simulink model "LoadFlow116BusNetwork_original"  (R2024a)
settings: Solver=FixedStepDiscrete  StartTime=0.0  StopTime=4.5  FixedStep=75e-6  RelTol=1e-3  EnableMultiTasking=on
undefined symbols (not defined in the file or in its folder): D1, D11, Delta
libraries: spsSeriesRLCBranchLib x164, spsLoadFlowBusLib x116, spsDistributedParametersLineLib x79, spsThreePhaseSeriesRLCLoadLib x60, spsThreePhaseTransformerTwoWindingsLib x52, spsThreePhaseParallelRLCLoadLib x44, spsThreePhaseVIMeasurementLib x44, spsSynchronousMachinepuStandardLib x28, spsExcitationSystemLib x28, spsHydraulicTurbineandGovernorLib x28, spsGenericPowerSystemStabilizerLib x28, spsMultiBandPowerSystemStabilizerLib x28
(part 5 of 15)

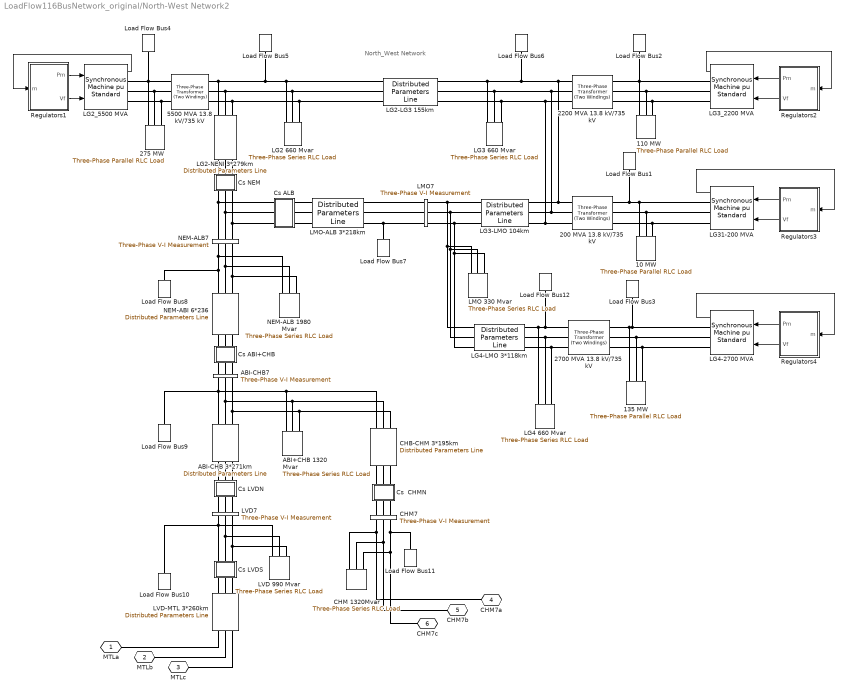
== system LoadFlow116BusNetwork_original/North-West Network2 ==
  note: North_West Network
  10 MW : spsThreePhaseParallelRLCLoadLib/Three-Phase Parallel RLC Load  LConnTagsString=A|B|C  Configuration=Y (grounded)  NominalVoltage=(13800)*1  Vabc=[1e3 1e3 1e3]  Vabcp=[1e3 1e3 1e3]  NominalFrequency=60  UnbalancedPower=off  ActivePower=10000000  InductivePower=0  CapacitivePower=0  Pabc=[10e3 9e3 11e3]  QLabc=[100 90 110]  QCabc=[100 90 110]  Pabcp=[10e3 9e3 11e3]  QLabcp=[100 90 110]  QCabcp=[100 90 110]  Measurements=None  LoadType=constant PQ
  110 MW : spsThreePhaseParallelRLCLoadLib/Three-Phase Parallel RLC Load  LConnTagsString=A|B|C  Configuration=Y (grounded)  NominalVoltage=(13800)*1  Vabc=[1e3 1e3 1e3]  Vabcp=[1e3 1e3 1e3]  NominalFrequency=60  UnbalancedPower=off  ActivePower=110000000  InductivePower=0  CapacitivePower=0  Pabc=[10e3 9e3 11e3]  QLabc=[100 90 110]  QCabc=[100 90 110]  Pabcp=[10e3 9e3 11e3]  QLabcp=[100 90 110]  QCabcp=[100 90 110]  Measurements=None  LoadType=constant PQ
  135 MW : spsThreePhaseParallelRLCLoadLib/Three-Phase Parallel RLC Load  LConnTagsString=A|B|C  Configuration=Y (grounded)  NominalVoltage=(13800)*1  Vabc=[1e3 1e3 1e3]  Vabcp=[1e3 1e3 1e3]  NominalFrequency=60  UnbalancedPower=off  ActivePower=135000000  InductivePower=0  CapacitivePower=0  Pabc=[10e3 9e3 11e3]  QLabc=[100 90 110]  QCabc=[100 90 110]  Pabcp=[10e3 9e3 11e3]  QLabcp=[100 90 110]  QCabcp=[100 90 110]  Measurements=None  LoadType=constant PQ
  200 MVA 13.8 kV/735 kV : spsThreePhaseTransformerTwoWindingsLib/Three-Phase Transformer (Two Windings)  Winding1Connection=Delta (D1)  Winding2Connection=Yg  CoreType=Three single-phase transformers  SetSaturation=off  Hysteresis=off  DataFile='basic_model'  SetInitialFlux=off  Measurements=None  UNITS=pu  NominalPower=[ 200e6 60 ]  Winding1="[ 13.8e3 0.002  0.0]"  Winding2=[ 735e3 0.002 0.12]  Rm=500  Lm=500  L0=0.5  Saturation="[ 0,0  ;  0.005,1.2  ;  1.0,1.4 ]"  InitialFluxes=[ 0.8 , -0.8 , 0.7 ]  BreakLoop=off  DiscreteSolver=Trapezoidal iterative  DataType=off  TransfoNumber=0
  2200 MVA 13.8 kV/735 kV : spsThreePhaseTransformerTwoWindingsLib/Three-Phase Transformer (Two Windings)  Winding1Connection=Delta (D1)  Winding2Connection=Yg  CoreType=Three single-phase transformers  SetSaturation=off  Hysteresis=off  DataFile='basic_model'  SetInitialFlux=off  Measurements=None  UNITS=pu  NominalPower=[ 2200e6 60 ]  Winding1="[ 13.8e3 0.002  0.0]"  Winding2=[ 735e3 0.002 0.12]  Rm=500  Lm=500  L0=0.5  Saturation="[ 0,0  ;  0.005,1.2  ;  1.0,1.4 ]"  InitialFluxes=[ 0.8 , -0.8 , 0.7 ]  BreakLoop=off  DiscreteSolver=Trapezoidal iterative  DataType=off  TransfoNumber=0
  2700 MVA 13.8 kV/735 kV : spsThreePhaseTransformerTwoWindingsLib/Three-Phase Transformer (Two Windings)  Winding1Connection=Delta (D1)  Winding2Connection=Yg  CoreType=Three single-phase transformers  SetSaturation=off  Hysteresis=off  DataFile='basic_model'  SetInitialFlux=off  Measurements=None  UNITS=pu  NominalPower=[ 2700e6 60 ]  Winding1="[ 13.8e3 0.002  0.0]"  Winding2=[ 735e3 0.002 0.12]  Rm=500  Lm=500  L0=0.5  Saturation="[ 0,0  ;  0.005,1.2  ;  1.0,1.4 ]"  InitialFluxes=[ 0.8 , -0.8 , 0.7 ]  BreakLoop=off  DiscreteSolver=Trapezoidal iterative  DataType=off  TransfoNumber=0
  275 MW : spsThreePhaseParallelRLCLoadLib/Three-Phase Parallel RLC Load  LConnTagsString=A|B|C  Configuration=Y (grounded)  NominalVoltage=(13800)*1  Vabc=[1e3 1e3 1e3]  Vabcp=[1e3 1e3 1e3]  NominalFrequency=60  UnbalancedPower=off  ActivePower=275000000  InductivePower=0  CapacitivePower=0  Pabc=[10e3 9e3 11e3]  QLabc=[100 90 110]  QCabc=[100 90 110]  Pabcp=[10e3 9e3 11e3]  QLabcp=[100 90 110]  QCabcp=[100 90 110]  Measurements=None  LoadType=constant PQ
  5500 MVA 13.8 kV/735 kV : spsThreePhaseTransformerTwoWindingsLib/Three-Phase Transformer (Two Windings)  Winding1Connection=Delta (D1)  Winding2Connection=Yg  CoreType=Three single-phase transformers  SetSaturation=off  Hysteresis=off  DataFile='basic_model'  SetInitialFlux=off  Measurements=None  UNITS=pu  NominalPower=[ 5500e6 60 ]  Winding1="[ 13.8e3 0.002  0.0]"  Winding2=[ 735e3 0.002 0.12]  Rm=500  Lm=500  L0=0.5  Saturation="[ 0,0  ;  0.005,1.2  ;  1.0,1.4 ]"  InitialFluxes=[ 0.8 , -0.8 , 0.7 ]  BreakLoop=off  DiscreteSolver=Trapezoidal iterative  DataType=off  TransfoNumber=0
  ABI+CHB 1320 Mvar : spsThreePhaseSeriesRLCLoadLib/Three-Phase Series RLC Load  LConnTagsString=A|B|C  Configuration=Y (grounded)  NominalVoltage=735e3  Vabc=[1e3 1e3 1e3]  Vabcp=[1e3 1e3 1e3]  NominalFrequency=60  UnbalancedPower=off  ActivePower=4400000  InductivePower=1320e6  CapacitivePower=0  Pabc=[10e3 9e3 11e3]  QLabc=[100 90 110]  QCabc=[100 90 110]  Pabcp=[10e3 9e3 11e3]  QLabcp=[100 90 110]  QCabcp=[100 90 110]  Measurements=None  LoadType=constant Z
  ABI-CHB 3*271km : spsDistributedParametersLineLib/Distributed Parameters Line  Phases=3  Length=271  Frequency=60  Resistance="[0.01273  0.3864]/3"  Inductance="[0.9337e-3  4.1264e-3]/3"  Capacitance=[12.74e-9 7.751e-9]*3  x1=[-0.001575 3.49112965554761e-09 -103484.456536088 -819305.847115511;-0.0015 3.54940703648419e-09 -80280.8596537815 -821903.919579572;-0.001425 3.60484707574356e-09 -57013.0874806064 -823844.974625874;-0.00135 3.65740545540659e-09 -33699.7399176288 -825127.46060471;-0.001275 3.70704016110874e-09 -10359.4532981844 -825750.352316412;-0.0012 3.75371151562572e-09 12989.1145097218 -825713.151830876;-0.001125 3.79738221059082e-09 36327.2990182289 -825015.888885602;-0.00105 3.83801733631867e-09 59636.4440397272 -823659.120861919;-0.000975 3.87558440971151e-09 82897.9166003282 -821643.932339426;-0.0009 3.91005340022564e-09 106093.12183478 -818971.934228995;-0.000825 3.94139675387747e-09 129203.517850916 -815645.262485032;-0.00075 3.96958941526963e-09 152210.630551762 -811666.57639803;-0.000675 3.99460884761998e-09 175096.068403445 -807039.05646877;-0.0006 4.01643505077712e-09 197841.537137107 -801766.40186588;-0.000525 4.03505057720817e-09 220428.854373058 -795852.827468776;-0.00045 4.05044054594615e-09 242839.964155498 -789303.06049835;-0.000375 4.06259265448552e-09 265056.951386168 -782122.336738104;-0.0003 4.07149718861665e-09 287062.056145408 -774316.396348742;-0.000225 4.07714703019119e-09 308837.687889161 -765891.479279577;-0.00015 4.07953766281224e-09 330366.439510591 -756854.320280409;-7.5e-05 4.07866717544465e-09 351631.101255053 -747212.143517868]  x2=[-0.001575 8.85627598143127e-09 -329701.158011524 -748762.187115691;-0.0015 9.00536203977742e-09 -308401.44100994 -757783.743021183;-0.001425 9.14724934949562e-09 -286855.192615113 -766199.538196984;-0.00135 9.28182448804145e-09 -265079.63656834 -774002.845185196;-0.001275 9.40897987810821e-09 -243092.179915949 -781187.426141608;-0.0012 9.52861387362263e-09 -220910.399094369 -787747.537822131;-0.001125 9.64063084099916e-09 -198552.025879795 -793677.93617386;-0.00105 9.74494123558799e-09 -176034.93321368 -798973.880527091;-0.000975 9.84146167325569e-09 -153377.12091538 -803631.13738494;-0.0009 9.93011499704121e-09 -130596.701293368 -807645.983807531;-0.000825 1.00108303388339e-08 -107711.884666539 -811015.210388065;-0.00075 1.00835431760247e-08 -84740.9648071545 -813736.123818364;-0.000675 1.01481953830838e-08 -61702.3043170834 -815806.549041862;-0.0006 1.02047352780264e-08 -38614.3199490181 -817224.830992315;-0.000525 1.02531176637254e-08 -15495.4678844046 -817989.835916832;-0.00045 1.02933038640419e-08 7635.77102014722 -818100.952282181;-0.000375 1.03252617547424e-08 30760.9060061767 -817558.09126364;-0.0003 1.03489657891779e-08 53861.4511946025 -816361.686816001;-0.000225 1.0364397018706e-08 76918.9403630512 -814512.695326674;-0.00015 1.0371543107838e-08 99914.9417074729 -812012.594851165;-7.5e-05 1.03703983440995e-08 122831.072576243 -808863.383931542]  x3=[-0.001575 -2.33509162895543e-12 -747.841433917336 -1501.46113433937;-0.0015 -8.83661713204438e-13 -705.09503694803 -1522.0023117976;-0.001425 5.68474588199612e-13 -661.784997794503 -1541.32682389519;-0.00135 2.02015645971581e-12 -617.94593783939 -1559.41922291285;-0.001275 3.47022344906753e-12 -573.612901356457 -1576.26504606363;-0.0012 4.91751639489027e-12 -528.821327496752 -1591.85082705425;-0.001125 6.36087835334746e-12 -483.607021959084 -1606.16410684986;-0.00105 7.79915552297369e-12 -438.006128367497 -1619.19344363358;-0.000975 9.23119816700594e-12 -392.055099378611 -1630.92842195296;-0.0009 1.06558615324655e-11 -345.790667541927 -1641.35966104587;-0.000825 1.20720067652562e-11 -299.249815936384 -1650.47882233938;-0.00075 1.34785018205467e-11 -252.469748606657 -1658.27861611549;-0.000675 1.48742223677098e-11 -205.487860822811 -1664.75280733839;-0.0006 1.62580526890954e-11 -158.341709187093 -1669.89622063867;-0.000525 1.76288865719179e-11 -111.06898161176 -1673.70474445044;-0.00045 1.89856281925458e-11 -63.7074671919388 -1676.17533429805;-0.000375 2.03271929924864e-11 -16.2950259976015 -1677.30601522975;-0.0003 2.16525085453653e-11 31.1304411911961 -1677.09588339653;-0.000225 2.29605154142075e-11 78.5310231816171 -1675.54510677455;-0.00015 2.42501679983353e-11 125.868828673672 -1672.65492503091;-7.5e-05 2.55204353692052e-11 173.106016549942 -1668.42764853267]  x4=[-0.001575 3.79881308339713e-11 -7080.29438162328 -14859.1258761626;-0.0015 3.76223755888515e-11 -6657.38891399992 -15053.3510061731;-0.001425 3.72265455923276e-11 -6229.16163154018 -15235.5427177132;-0.00135 3.68009572648424e-11 -5795.95485258156 -15405.5553695164;-0.001275 3.63459508151933e-11 -5358.11487599487 -15563.2530560702;-0.0012 3.58618899685742e-11 -4915.99170435821 -15708.5097162566;-0.001125 3.53491616758195e-11 -4469.93876417028 -15841.2092341242;-0.00105 3.48081758040815e-11 -4020.31262332663 -15961.2455317086;-0.000975 3.42393648091886e-11 -3567.47270608474 -16068.5226538302;-0.0009 3.36431833899472e-11 -3111.78100574577 -16162.9548447989;-0.000825 3.30201081246617e-11 -2653.60179528266 -16244.4666169663;-0.00075 3.23706370901661e-11 -2193.30133614586 -16312.9928110687;-0.000675 3.16952894636679e-11 -1731.24758547958 -16368.4786483151;-0.0006 3.09946051077266e-11 -1267.80990198245 -16410.8797741762;-0.000525 3.02691441386956e-11 -803.358750647814 -16440.1622938406;-0.00045 2.95194864789735e-11 -338.265406619711 -16456.3027993103;-0.000375 2.87462313934234e-11 127.098341598809 -16459.2883881121;-0.0003 2.79499970103296e-11 592.360489347724 -16449.116673612;-0.000225 2.71314198272749e-11 1057.14911318487 -16425.795786923;-0.00015 2.6291154202335e-11 1521.09266819587 -16389.3443704049;-7.5e-05 2.54298718309939e-11 1983.82028500141 -16339.7915627626]  x5=0.00153261764655846  V1=ones(3,3)  V2=ones(3,3)  I1=ones(3,3)  I2=ones(3,3)  nHarmo=1  Measurements=None  Decoupling=off  VsMag0=[ 1 1 1]  VrMag0=[ 1 1 1]  VsAngle0=[0 -120 120]  VrAngle0=[0 -120 120]  IsMag0=[ 1 1 1]  IrMag0=[ 1 1 1]  IsAngle0=[0 -120 120]  IrAngle0=[0 -120 120]
      settings: AttributesFormatString=\n  LibrarySourceBlock=sps_lib/Power Grid Elements/Distributed Parameters Line
  ABI-CHB7 : spsThreePhaseVIMeasurementLib/Three-Phase V-I Measurement  VoltageMeasurement=no  SetLabelV=on  LabelV=Vabc_ABI7  Vpu=on  VpuLL=off  CurrentMeasurement=no  SetLabelI=off  LabelI=A1  Ipu=off  Pbase=100e6  Vbase=500e3  OutputType=Magnitude  PhasorSimulation=off  PSBequivalent=0
  CHB-CHM 3*195km : spsDistributedParametersLineLib/Distributed Parameters Line  Phases=3  Length=195  Frequency=60  Resistance="[0.01273  0.3864]/3"  Inductance="[0.9337e-3  4.1264e-3]/3"  Capacitance=[12.74e-9 7.751e-9]*3  x1=[-0.001125 3.79738221059082e-09 0 0;-0.00105 3.83801733631867e-09 0 0;-0.000975 3.87558440971151e-09 0 0;-0.0009 3.91005340022564e-09 0 0;-0.000825 3.94139675387747e-09 0 0;-0.00075 3.96958941526963e-09 0 0;-0.000675 3.99460884761998e-09 175096.068403445 -807039.05646877;-0.0006 4.01643505077712e-09 197841.537137107 -801766.40186588;-0.000525 4.03505057720817e-09 220428.854373058 -795852.827468776;-0.00045 4.05044054594615e-09 242839.964155498 -789303.06049835;-0.000375 4.06259265448552e-09 265056.951386168 -782122.336738104;-0.0003 4.07149718861665e-09 287062.056145408 -774316.396348742;-0.000225 4.07714703019119e-09 308837.687889161 -765891.479279577;-0.00015 4.07953766281224e-09 330366.439510591 -756854.320280409;-7.5e-05 4.07866717544465e-09 351631.101255053 -747212.143517868]  x2=[-0.001125 2.70727178831933e-09 0 0;-0.00105 2.73262221708917e-09 0 0;-0.000975 2.75578822946918e-09 0 0;-0.0009 2.77675130690354e-09 0 0;-0.000825 2.79549469182887e-09 0 0;-0.00075 2.81200340107006e-09 0 0;-0.000675 2.82626423781753e-09 86661.6913681537 -814290.344127287;-0.0006 2.83826580217658e-09 109647.510746712 -811514.902082689;-0.000525 2.8479985002803e-09 132545.679582843 -808090.747441961;-0.00045 2.85545455195872e-09 155337.893430733 -804020.617421931;-0.000375 2.86062799695824e-09 178005.932543363 -799307.765622262;-0.0003 2.86351469970606e-09 200531.6764371 -793955.959424573;-0.000225 2.86411235261617e-09 222897.118376931 -787969.476980854;-0.00015 2.862420477934e-09 245084.379770771 -781353.103793574;-7.5e-05 2.85844042811827e-09 267075.72446134 -774112.128890224]  x3=[-0.001125 1.76155641183731e-11 0 0;-0.00105 1.7454951833372e-11 0 0;-0.000975 1.72803863269451e-11 0 0;-0.0009 1.70920071440872e-11 0 0;-0.000825 1.68899648722348e-11 0 0;-0.00075 1.66744210208886e-11 0 0;-0.000675 1.64455478925056e-11 335.259499976979 -5255.16303225153;-0.0006 1.62035284447626e-11 483.69285157656 -5243.58412650834;-0.000525 1.59485561443032e-11 631.73954651134 -5227.81357984395;-0.00045 1.5680834812083e-11 779.281238518578 -5207.86399899206;-0.000375 1.5400578460439e-11 926.199985027146 -5183.75133134236;-0.0003 1.51080111220104e-11 1072.37834143902 -5155.49485219245;-0.000225 1.48033666706512e-11 1217.69945501268 -5123.11714933941;-0.00015 1.44868886344746e-11 1362.04715827344 -5086.64410502351;-7.5e-05 1.41588300011804e-11 1505.30606187589 -5046.10487523831]  x4=[-0.001125 5.67670866959794e-12 0 0;-0.00105 6.209051937135e-12 0 0;-0.000975 6.73643178355519e-12 0 0;-0.0009 7.25842662947847e-12 0 0;-0.000825 7.7746192002118e-12 0 0;-0.00075 8.28459685931214e-12 0 0;-0.000675 8.78795193844173e-12 265.942029614519 -12956.0177279487;-0.0006 9.2842820632519e-12 632.108856781867 -12943.3211843342;-0.000525 9.77319047503499e-12 997.770385800693 -12920.2779478045;-0.00045 1.02542863478872e-11 1362.63431243951 -12886.9064387702;-0.000375 1.07271851011287e-11 1726.40897005797 -12843.2333339049;-0.0003 1.11915087067318e-11 2088.8035627607 -12789.2935448207;-0.000225 1.16468859915106e-11 2449.52839785513 -12725.1301901594;-0.00015 1.20929529338311e-11 2808.29511742736 -12650.7945611252;-7.5e-05 1.25293529546046e-11 3164.81692885107 -12566.3460804824]  x5=0.0011028060556417  V1=ones(3,3)  V2=ones(3,3)  I1=ones(3,3)  I2=ones(3,3)  nHarmo=1  Measurements=None  Decoupling=off  VsMag0=[ 1 1 1]  VrMag0=[ 1 1 1]  VsAngle0=[0 -120 120]  VrAngle0=[0 -120 120]  IsMag0=[ 1 1 1]  IrMag0=[ 1 1 1]  IsAngle0=[0 -120 120]  IrAngle0=[0 -120 120]
      settings: AttributesFormatString=\n  LibrarySourceBlock=sps_lib/Power Grid Elements/Distributed Parameters Line
  CHM 1320Mvar : spsThreePhaseSeriesRLCLoadLib/Three-Phase Series RLC Load  LConnTagsString=A|B|C  Configuration=Y (grounded)  NominalVoltage=735e3  Vabc=[1e3 1e3 1e3]  Vabcp=[1e3 1e3 1e3]  NominalFrequency=60  UnbalancedPower=off  ActivePower=4400000  InductivePower=1320e6  CapacitivePower=0  Pabc=[10e3 9e3 11e3]  QLabc=[100 90 110]  QCabc=[100 90 110]  Pabcp=[10e3 9e3 11e3]  QLabcp=[100 90 110]  QCabcp=[100 90 110]  Measurements=None  LoadType=constant Z
  CHM7 : spsThreePhaseVIMeasurementLib/Three-Phase V-I Measurement  VoltageMeasurement=no  SetLabelV=on  LabelV=Vabc_CHM7  Vpu=on  VpuLL=off  CurrentMeasurement=no  SetLabelI=off  LabelI=A1  Ipu=off  Pbase=100e6  Vbase=735e3  OutputType=Magnitude  PhasorSimulation=off  PSBequivalent=0
  "Cs  CHMN " : Subsystem  mask{Xc=25/3}
      mask prompts: Xc "Condensator Reactance at  60Hz  (ohm):"
      mask help: Series Compensation
      mask init:
      | Cs=1/Xc/(2*pi*60);
      mask Display: disp('Cs')
  "Cs ABI+CHB " : Subsystem  mask{Xc=25/6}
      mask prompts: Xc "Condensator Reactance at  60Hz  (ohm):"
      mask help: Series Compensation
      mask init:
      | Cs=1/Xc/(2*pi*60);
      mask Display: disp('Cs')
  Cs ALB : Subsystem  mask{Xc=16/3}
      mask prompts: Xc "Reactance @ 60Hz du condensateur (ohm):"
      mask init:
      | Cs=1/Xc/(2*pi*60);
      mask Display: disp('Cs')
  "Cs LVDN " : Subsystem  mask{Xc=34/3}
      mask prompts: Xc "Condensator Reactance at  60Hz  (ohm):"
      mask help: Series Compensation
      mask init:
      | Cs=1/Xc/(2*pi*60);
      mask Display: disp('Cs')
  "Cs LVDS " : Subsystem  mask{Xc=34/3}
      mask prompts: Xc "Condensator Reactance at  60Hz  (ohm):"
      mask help: Series Compensation
      mask init:
      | Cs=1/Xc/(2*pi*60);
      mask Display: disp('Cs')
  "Cs NEM " : Subsystem  mask{Xc=16/3}
      mask prompts: Xc "Condensator Reactance at  60Hz  (ohm):"
      mask help: Series Compensation
      mask init:
      | Cs=1/Xc/(2*pi*60);
      mask Display: disp('Cs')
  LG2 660 Mvar : spsThreePhaseSeriesRLCLoadLib/Three-Phase Series RLC Load  LConnTagsString=A|B|C  Configuration=Y (grounded)  NominalVoltage=735e3  Vabc=[1e3 1e3 1e3]  Vabcp=[1e3 1e3 1e3]  NominalFrequency=60  UnbalancedPower=off  ActivePower=2200000  InductivePower=660e6  CapacitivePower=0  Pabc=[10e3 9e3 11e3]  QLabc=[100 90 110]  QCabc=[100 90 110]  Pabcp=[10e3 9e3 11e3]  QLabcp=[100 90 110]  QCabcp=[100 90 110]  Measurements=None  LoadType=constant Z
  LG2-LG3 155km : spsDistributedParametersLineLib/Distributed Parameters Line  Phases=3  Length=155  Frequency=60  Resistance="[0.01273  0.3864]"  Inductance="[0.9337e-3  4.1264e-3]"  Capacitance=[12.74e-9 7.751e-9]  x1=[-0.0009 -6.87729294283737e-10 371984.249881849 -674633.962928184;-0.000825 -6.47200167873324e-10 390907.835511781 -663848.0492385;-0.00075 -6.06153679551209e-10 409518.935399095 -652531.465575472;-0.000675 -5.64622641252122e-10 427802.672115301 -640693.258242928;-0.0006 -5.22640252252635e-10 445744.429921019 -628342.890522681;-0.000525 -4.8024007263216e-10 463329.866449576 -615490.235109718;-0.00045 -4.37455996445544e-10 480544.924172078 -602145.566220125;-0.000375 -3.94322224628669e-10 497375.841634781 -588319.551378032;-0.0003 -3.50873237658759e-10 513809.164459787 -574023.242888158;-0.000225 -3.07143767991206e-10 529831.756100267 -559268.06900077;-0.00015 -2.63168772294977e-10 545430.808341618 -544065.824776111;-7.5e-05 -2.18983403508793e-10 560593.851540153 -528428.662655612]  x2=[-0.0009 -7.31319823534682e-10 375373.731714456 -666225.89635668;-0.000825 -7.83695746758994e-10 394058.262242389 -655347.523812972;-0.00075 -8.35445195594294e-10 412427.78862478 -643945.276485881;-0.000675 -8.86526802322976e-10 430467.6265433 -632028.26915746;-0.0006 -9.36899733090196e-10 448163.355227538 -619606.028101032;-0.000525 -9.8652372054583e-10 465500.828982735 -606688.48346603;-0.00045 -1.03535909603358e-09 482466.188497646 -593285.96133999;-0.000375 -1.08336682130148e-09 499045.871923451 -579409.175494035;-0.0003 -1.13050851970851e-09 515226.625714899 -565069.218818447;-0.000225 -1.17674650690224e-09 530995.515224982 -550277.554455185;-0.00015 -1.22204382094318e-09 546339.935044698 -535046.00663442;-7.5e-05 -1.26636425185155e-09 561247.619079621 -519386.75122243]  x3=[-0.0009 1.13728235254083e-11 1272.11889165594 -2673.50704029698;-0.000825 1.13378200724857e-11 1347.1919564629 -2636.47471081206;-0.00075 1.12937533396716e-11 1421.1880966326 -2597.33482378272;-0.000675 1.1240658553238e-11 1494.04816078275 -2556.11866703581;-0.0006 1.11785781563448e-11 1565.71390569288 -2512.8591881364;-0.000525 1.11075617751113e-11 1636.12804286303 -2467.59096805002;-0.00045 1.10276661789463e-11 1705.2342843093 -2420.3501934992;-0.000375 1.09389552351667e-11 1772.97738755966 -2371.17462803629;-0.0003 1.08414998579438e-11 1839.30319981387 -2320.10358185592;-0.000225 1.07353779516149e-11 1904.15870123243 -2267.17788037099;-0.00015 1.06206743484083e-11 1967.49204731983 -2212.43983157747;-7.5e-05 1.04974807406294e-11 2029.25261036824 -2155.93319223405]  x4=[-0.0009 -1.58214802470238e-11 974.452643997904 -2530.47846704095;-0.000825 -1.57898319315028e-11 1045.60107405625 -2501.9185223219;-0.00075 -1.57455614659282e-11 1115.91366661423 -2471.35858221674;-0.000675 -1.5688704239433e-11 1185.33421486118 -2438.82307587402;-0.0006 -1.5619305702814e-11 1253.80722507298 -2404.33801167968;-0.000525 -1.55374213321996e-11 1321.27796097295 -2367.93095646641;-0.00045 -1.54431165847027e-11 1387.69248748716 -2329.6310134771;-0.000375 -1.53364668460956e-11 1452.99771385927 -2289.46879910017;-0.0003 -1.52175573705476e-11 1517.14143609053 -2247.47641839528;-0.000225 -1.5086483212474e-11 1580.07237867083 -2203.68743942907;-0.00015 -1.49433491505512e-11 1641.74023556754 -2158.13686644133;-7.5e-05 -1.47882696039584e-11 1702.0957104394 -2110.86111186316]  x5=0.000876589428843401  V1=ones(3,3)  V2=ones(3,3)  I1=ones(3,3)  I2=ones(3,3)  nHarmo=1  Measurements=None  Decoupling=off  VsMag0=[ 1 1 1]  VrMag0=[ 1 1 1]  VsAngle0=[0 -120 120]  VrAngle0=[0 -120 120]  IsMag0=[ 1 1 1]  IrMag0=[ 1 1 1]  IsAngle0=[0 -120 120]  IrAngle0=[0 -120 120]
      settings: AttributesFormatString=\n  LibrarySourceBlock=sps_lib/Power Grid Elements/Distributed Parameters Line
  LG2-NENI 3*279km : spsDistributedParametersLineLib/Distributed Parameters Line  Phases=3  Length=279  Frequency=60  Resistance="[0.01273  0.3864]/3"  Inductance="[0.9337e-3  4.1264e-3]/3"  Capacitance=[12.74e-9 7.751e-9]*3  x1=[-0.00165 -1.05767542521649e-09 168997.444324008 -751627.644710185;-0.001575 -1.02402106564683e-09 190178.800707055 -746549.517209765;-0.0015 -9.89548119305339e-10 211208.131066651 -740874.609447879;-0.001425 -9.54284143337871e-10 232068.624877864 -734607.457858961;-0.00135 -9.18257327227255e-10 252743.606581119 -727753.072308102;-0.001275 -8.81496470259063e-10 273216.548912379 -720316.932086236;-0.0012 -8.44030958499893e-10 293471.086114793 -712304.981530078;-0.001125 -8.05890741306606e-10 313491.027021224 -703723.625270317;-0.00105 -7.67106307385259e-10 333260.367997229 -694579.723111847;-0.000975 -7.27708660418909e-10 352763.305734111 -684880.584550148;-0.0009 -6.87729294283736e-10 371984.249881849 -674633.962928184;-0.000825 -6.47200167873324e-10 390907.835511781 -663848.0492385;-0.00075 -6.06153679551208e-10 409518.935399095 -652531.465575472;-0.000675 -5.64622641252122e-10 427802.672115301 -640693.258242928;-0.0006 -5.22640252252635e-10 445744.429921019 -628342.890522681;-0.000525 -4.8024007263216e-10 463329.866449576 -615490.235109718;-0.00045 -4.37455996445544e-10 480544.924172078 -602145.566220125;-0.000375 -3.94322224628669e-10 497375.841634781 -588319.551378032;-0.0003 -3.50873237658759e-10 513809.164459787 -574023.242888158;-0.000225 -3.07143767991206e-10 529831.756100267 -559268.06900077;-0.00015 -2.63168772294977e-10 545430.808341618 -544065.824776111;-7.5e-05 -2.18983403508793e-10 560593.851540153 -528428.662655612]  x2=[-0.00165 1.84310759312133e-09 -47534.3064646231 -809002.983106273;-0.001575 1.90807753271091e-09 -24644.3461224049 -810023.42622981;-0.0015 1.97152218431542e-09 -1734.68546696752 -810396.349020192;-0.001425 2.03339083125108e-09 21176.3618694905 -810121.453368647;-0.00135 2.09363401666816e-09 44070.4811462793 -809198.959022554;-0.001275 2.15220358308599e-09 66929.3711547407 -807629.603409777;-0.0012 2.20905271088932e-09 89734.7588479548 -805414.641049181;-0.001125 2.26413595575521e-09 112468.413947934 -802555.842547789;-0.00105 2.31740928498051e-09 135112.163518627 -799055.493185379;-0.000975 2.36883011268094e-09 157647.906493089 -794916.391087676;-0.0009 2.41835733383362e-09 180057.628143194 -790141.844989567;-0.000825 2.46595135713573e-09 202323.414480336 -784735.671590148;-0.00075 2.51157413665327e-09 224427.466575594 -778702.192501719;-0.000675 2.55518920223435e-09 246352.114787927 -772046.230795146;-0.0006 2.59676168866286e-09 268079.832889012 -764773.10714438;-0.000525 2.63625836352925e-09 289593.252073445 -756888.635573183;-0.00045 2.67364765379593e-09 310875.174843095 -748399.118807494;-0.000375 2.70889967103635e-09 331908.588754526 -739311.34323712;-0.0003 2.7419862353273e-09 352676.680018478 -729632.573490806;-0.000225 2.77288089777553e-09 373162.846940557 -719370.546628995;-0.00015 2.80155896166057e-09 393350.713192376 -708533.465958948;-7.5e-05 2.82799750217695e-09 413224.140902536 -697129.994477139]  x3=[-0.00165 -7.8460552892061e-12 -1677.04894976774 -1941.35400834287;-0.001575 -7.2159373400927e-12 -1621.4950861715 -1987.98793711402;-0.0015 -6.58005108107717e-12 -1564.64502421308 -2033.03269874547;-0.001425 -5.93890482990559e-12 -1506.54420896217 -2076.45228514399;-0.00135 -5.29301110908128e-12 -1447.23908532153 -2118.21198735655;-0.001275 -4.64288623616215e-12 -1386.77706089957 -2158.27842331615;-0.0012 -3.98904991102437e-12 -1325.20646811354 -2196.61956452691;-0.001125 -3.33202480042224e-12 -1262.57652555323 -2233.2047616672;-0.00105 -2.67233612017633e-12 -1198.93729863646 -2268.00476909019;-0.000975 -2.01051121532407e-12 -1134.33965958752 -2300.99176820241;-0.0009 -1.34707913856813e-12 -1068.83524677069 -2332.13938970148;-0.000825 -6.82570227359823e-13 -1002.47642341131 -2361.42273465535;-0.00075 -1.75156799554388e-14 -935.316235737464 -2388.81839440612;-0.000675 6.47552869215505e-13 -867.408370575585 -2414.30446928255;-0.0006 1.31210377453069e-12 -798.807112434063 -2437.86058610633;-0.000525 1.97560580416437e-12 -729.567300109018 -2459.46791447809;-0.00045 2.63752856474599e-12 -659.744282847021 -2479.10918183014;-0.000375 3.29734292534849e-12 -589.393876099742 -2496.76868723388;-0.0003 3.9545214404675e-12 -518.572316905937 -2512.43231395089;-0.000225 4.60853877165321e-12 -447.336218936421 -2526.08754071763;-0.00015 5.25887210745787e-12 -375.74252723796 -2537.72345175475;-7.5e-05 5.90500158136327e-12 -303.848472712279 -2547.33074549301]  x4=[-0.00165 6.20428474912396e-12 -141.249463960485 -15427.0315937085;-0.001575 5.91618923955736e-12 294.93685075288 -15424.8591939206;-0.0015 5.62336441883339e-12 730.887397460438 -15410.3563977013;-0.001425 5.32604436663336e-12 1166.25368396542 -15383.534798364;-0.00135 5.02446675605785e-12 1600.68768511972 -15344.4158366849;-0.001275 4.71887266363448e-12 2033.84212102987 -15293.0307837634;-0.0012 4.40950637660497e-12 2465.37073466731 -15229.4207160246;-0.001125 4.09661519764571e-12 2894.92856866088 -15153.6364823833;-0.00105 3.78044924717776e-12 3322.17224105057 -15065.7386635965;-0.000975 3.46126126342443e-12 3746.76021978169 -14965.7975238355;-0.0009 3.1393064003762e-12 4168.35309572048 -14853.8929545183;-0.000825 2.81484202382451e-12 4586.61385397249 -14730.1144104454;-0.00075 2.48812750562749e-12 5001.20814328717 -14594.5608382912;-0.000675 2.15942401637211e-12 5411.80454333317 -14447.340597507;-0.0006 1.82899431659833e-12 5818.07482963061 -14288.571373701;-0.000525 1.49710254675242e-12 6219.69423592877 -14118.3800845613;-0.00045 1.16401401603706e-12 6616.34171381925 -13936.9027784005;-0.000375 8.29994990327305e-13 7007.70018937712 -13744.2845254003;-0.0003 4.95312479321627e-13 7393.45681662501 -13540.6793016452;-0.000225 1.60234023098514e-13 7773.30322761738 -13326.2498660357;-0.00015 -1.74972521751001e-13 8146.93577894511 -13101.1676301817;-7.5e-05 -5.10039196243798e-13 8514.05579446346 -12865.6125213788]  x5=0.00157786097191812  V1=ones(3,3)  V2=ones(3,3)  I1=ones(3,3)  I2=ones(3,3)  nHarmo=1  Measurements=None  Decoupling=off  VsMag0=[ 1 1 1]  VrMag0=[ 1 1 1]  VsAngle0=[0 -120 120]  VrAngle0=[0 -120 120]  IsMag0=[ 1 1 1]  IrMag0=[ 1 1 1]  IsAngle0=[0 -120 120]  IrAngle0=[0 -120 120]
      settings: AttributesFormatString=\n  LibrarySourceBlock=sps_lib/Power Grid Elements/Distributed Parameters Line
  LG2_5500 MVA : spsSynchronousMachinepuStandardLib/Synchronous Machine pu Standard  PresetModel=No  MechanicalLoad=Mechanical power Pm  ShowDetailedParameters=on  RotorType=Salient-pole  Units=per unit standard parameters  MeasurementBus=off  NominalParameters="[5500E6  13800   60 ]"  Reactances1=[ 31 32 33 34 35 36 37 ]  Reactances2=[ 1.305, 0.296, 0.252, 0.474, 0.243, 0.18 ]  dAxisTimeConstants=Short-circuit  qAxisTimeConstants=Open-circuit  TimeConstants1=[]  TimeConstants2=[]  TimeConstants3=[]  TimeConstants4=[]  TimeConstants5=[ 1.01, 0.053, 0.1 ]  TimeConstants6=[]  TimeConstants7=[]  TimeConstants8=[]  StatorResistance=2.8544e-3  Mechanical="[ 4.1  0  32]"  PolePairs=32  InitialConditions=[0 -65.2434 0.985682 0.985682 0.985682 -1.22427 -121.224 118.776 1.47412]  SetSaturation=off  Saturation=[0.6404,0.7127,0.8441,0.9214,0.9956,1.082,1.19,1.316,1.457;0.7,0.7698,0.8872,0.9466,0.9969,1.046,1.1,1.151,1.201]  LoadFlowParameters=[2 4000000000 0 0 0]  TsPowergui=0  TsBlock=-1  IterativeModel=Trapezoidal non iterative  IterativeDiscreteModel=Trapezoidal non iterative  BusType=swing  Pref=0  Qref=0  Qmin=-Inf  Qmax=Inf  PLF=0  QLF=0
  LG3 660 Mvar : spsThreePhaseSeriesRLCLoadLib/Three-Phase Series RLC Load  LConnTagsString=A|B|C  Configuration=Y (grounded)  NominalVoltage=735e3  Vabc=[1e3 1e3 1e3]  Vabcp=[1e3 1e3 1e3]  NominalFrequency=60  UnbalancedPower=off  ActivePower=2200000  InductivePower=660e6  CapacitivePower=0  Pabc=[10e3 9e3 11e3]  QLabc=[100 90 110]  QCabc=[100 90 110]  Pabcp=[10e3 9e3 11e3]  QLabcp=[100 90 110]  QCabcp=[100 90 110]  Measurements=None  LoadType=constant Z
  LG3-LMO 104km : spsDistributedParametersLineLib/Distributed Parameters Line  Phases=3  Length=104  Frequency=60  Resistance="[0.01273  0.3864]"  Inductance="[0.9337e-3  4.1264e-3]"  Capacitance=[12.74e-9 7.751e-9]  x1=[-0.0006 -8.9322907973412e-10 0 0;-0.000525 -9.40897824308649e-10 0 0;-0.00045 -9.87814429558645e-10 0 0;-0.000375 -1.03394139106772e-09 499045.871923451 -579409.175494035;-0.0003 -1.07924183564861e-09 515226.625714899 -565069.218818447;-0.000225 -1.12367955081903e-09 530995.515224982 -550277.554455185;-0.00015 -1.16721901374941e-09 546339.935044698 -535046.00663442;-7.5e-05 -1.20982541965924e-09 561247.619079621 -519386.75122243]  x2=[-0.0006 5.23109448259394e-10 0 0;-0.000525 5.02663633370164e-10 0 0;-0.00045 4.81815996863429e-10 0 0;-0.000375 4.60583204020834e-10 445735.71370684 -651849.764162748;-0.0003 4.38982228012103e-10 463985.717973781 -638987.984734845;-0.000225 4.17030336326953e-10 481864.819156992 -625615.408088788;-0.00015 3.94745076971722e-10 499358.724976549 -611742.724057743;-7.5e-05 3.72144264441761e-10 516453.451071804 -597381.022253063]  x3=[-0.0006 -5.28597489983234e-12 0 0;-0.000525 -5.05275632097683e-12 0 0;-0.00045 -4.81549864602809e-12 0 0;-0.000375 -4.57439153514132e-12 -337.815764584116 -872.913223711312;-0.0003 -4.3296277256519e-12 -313.002403558299 -882.1141951894;-0.000225 -4.08140287800412e-12 -287.938833200174 -890.610018076654;-0.00015 -3.82991541934321e-12 -262.645088944402 -898.393900942247;-7.5e-05 -3.57536638489576e-12 -237.141390223131 -905.459621469315]  x4=[-0.0006 1.8679767955248e-12 0 0;-0.000525 1.60987638655869e-12 0 0;-0.00045 1.35048906704109e-12 0 0;-0.000375 1.09002218722649e-12 3507.69484614616 -3894.26054707415;-0.0003 8.28683960353307e-13 3616.38515846598 -3793.53952688977;-0.000225 5.66683296201511e-13 3722.18458782268 -3689.7860092507;-0.00015 3.04229634093278e-13 3825.00855977121 -3583.08293313145;-7.5e-05 4.15327754704193e-14 3924.77487840165 -3473.51559533847]  x5=0.000588163229675572  V1=ones(3,3)  V2=ones(3,3)  I1=ones(3,3)  I2=ones(3,3)  nHarmo=1  Measurements=None  Decoupling=off  VsMag0=[ 1 1 1]  VrMag0=[ 1 1 1]  VsAngle0=[0 -120 120]  VrAngle0=[0 -120 120]  IsMag0=[ 1 1 1]  IrMag0=[ 1 1 1]  IsAngle0=[0 -120 120]  IrAngle0=[0 -120 120]
      settings: AttributesFormatString=\n  LibrarySourceBlock=sps_lib/Power Grid Elements/Distributed Parameters Line
  LG31-200 MVA : spsSynchronousMachinepuStandardLib/Synchronous Machine pu Standard  PresetModel=No  MechanicalLoad=Mechanical power Pm  ShowDetailedParameters=on  RotorType=Salient-pole  Units=per unit standard parameters  MeasurementBus=off  NominalParameters="[200E6  13800   60 ]"  Reactances1=[ 31 32 33 34 35 36 37 ]  Reactances2=[ 1.305, 0.296, 0.252, 0.474, 0.243, 0.18 ]  dAxisTimeConstants=Short-circuit  qAxisTimeConstants=Open-circuit  TimeConstants1=[]  TimeConstants2=[]  TimeConstants3=[]  TimeConstants4=[]  TimeConstants5=[ 1.01, 0.053, 0.1 ]  TimeConstants6=[]  TimeConstants7=[]  TimeConstants8=[]  StatorResistance=2.8544e-3  Mechanical="[ 3.2  0  32]"  PolePairs=32  InitialConditions=[0 -67.6291 0.902477 0.902477 0.902477 -4.2812 -124.281 115.719 1.45511]  SetSaturation=off  Saturation=[0.6404,0.7127,0.8441,0.9214,0.9956,1.082,1.19,1.316,1.457;0.7,0.7698,0.8872,0.9466,0.9969,1.046,1.1,1.151,1.201]  LoadFlowParameters=[1 180000000 0 0 0]  TsPowergui=0  TsBlock=-1  IterativeModel=Trapezoidal non iterative  IterativeDiscreteModel=Trapezoidal non iterative  BusType=PV  Pref=180000000  Qref=0  Qmin=-Inf  Qmax=Inf  PLF=0  QLF=0
  LG3_2200 MVA : spsSynchronousMachinepuStandardLib/Synchronous Machine pu Standard  PresetModel=No  MechanicalLoad=Mechanical power Pm  ShowDetailedParameters=on  RotorType=Salient-pole  Units=per unit standard parameters  MeasurementBus=off  NominalParameters="[2200E6  13800   60 ]"  Reactances1=[ 31 32 33 34 35 36 37 ]  Reactances2=[ 1.305, 0.296, 0.252, 0.474, 0.243, 0.18 ]  dAxisTimeConstants=Short-circuit  qAxisTimeConstants=Open-circuit  TimeConstants1=[]  TimeConstants2=[]  TimeConstants3=[]  TimeConstants4=[]  TimeConstants5=[ 1.01, 0.053, 0.1 ]  TimeConstants6=[]  TimeConstants7=[]  TimeConstants8=[]  StatorResistance=2.8544e-3  Mechanical="[ 3.2  0  32]"  PolePairs=32  InitialConditions=[0 -70.0065 0.820496 0.820496 0.820496 -4.90643 -124.906 115.094 1.38903]  SetSaturation=off  Saturation=[0.6404,0.7127,0.8441,0.9214,0.9956,1.082,1.19,1.316,1.457;0.7,0.7698,0.8872,0.9466,0.9969,1.046,1.1,1.151,1.201]  LoadFlowParameters=[1 1800000000 0 0 0]  TsPowergui=0  TsBlock=-1  IterativeModel=Trapezoidal non iterative  IterativeDiscreteModel=Trapezoidal non iterative  BusType=PV  Pref=1800000000  Qref=0  Qmin=-Inf  Qmax=Inf  PLF=0  QLF=0
  LG4 660 Mvar : spsThreePhaseSeriesRLCLoadLib/Three-Phase Series RLC Load  LConnTagsString=A|B|C  Configuration=Y (grounded)  NominalVoltage=735e3  Vabc=[1e3 1e3 1e3]  Vabcp=[1e3 1e3 1e3]  NominalFrequency=60  UnbalancedPower=off  ActivePower=2200000  InductivePower=660e6  CapacitivePower=0  Pabc=[10e3 9e3 11e3]  QLabc=[100 90 110]  QCabc=[100 90 110]  Pabcp=[10e3 9e3 11e3]  QLabcp=[100 90 110]  QCabcp=[100 90 110]  Measurements=None  LoadType=constant Z
  LG4-2700 MVA : spsSynchronousMachinepuStandardLib/Synchronous Machine pu Standard  PresetModel=No  MechanicalLoad=Mechanical power Pm  ShowDetailedParameters=on  RotorType=Salient-pole  Units=per unit standard parameters  MeasurementBus=off  NominalParameters="[2700E6  13800   60 ]"  Reactances1=[ 31 32 33 34 35 36 37 ]  Reactances2=[ 1.305, 0.296, 0.252, 0.474, 0.243, 0.18 ]  dAxisTimeConstants=Short-circuit  qAxisTimeConstants=Open-circuit  TimeConstants1=[]  TimeConstants2=[]  TimeConstants3=[]  TimeConstants4=[]  TimeConstants5=[ 1.01, 0.053, 0.1 ]  TimeConstants6=[]  TimeConstants7=[]  TimeConstants8=[]  StatorResistance=2.8544e-3  Mechanical="[ 3.7  0  32]"  PolePairs=32  InitialConditions=[0 -69.506 0.926038 0.926038 0.926038 -2.40174 -122.402 117.598 1.38766]  SetSaturation=off  Saturation=[0.6404,0.7127,0.8441,0.9214,0.9956,1.082,1.19,1.316,1.457;0.7,0.7698,0.8872,0.9466,0.9969,1.046,1.1,1.151,1.201]  LoadFlowParameters=[1 2500000000 0 0 0]  TsPowergui=0  TsBlock=-1  IterativeModel=Trapezoidal non iterative  IterativeDiscreteModel=Trapezoidal non iterative  BusType=PV  Pref=2500000000  Qref=0  Qmin=-Inf  Qmax=Inf  PLF=0  QLF=0
  LG4-LMO 3*118km : spsDistributedParametersLineLib/Distributed Parameters Line  Phases=3  Length=118  Frequency=60  Resistance="[0.01273  0.3864]/3"  Inductance="[0.9337e-3  4.1264e-3]/3"  Capacitance=[12.74e-9 7.751e-9]*3  x1=[-0.000675 -1.0685468036217e-09 400494.98918038 -665247.597360501;-0.0006 -1.10233210023585e-09 419141.837998236 -653659.450927313;-0.000525 -1.13523620943531e-09 437453.631243882 -641548.77913038;-0.00045 -1.16723282817865e-09 455415.730749976 -628925.263055435;-0.000375 -1.1982963788584e-09 473013.777889002 -615798.993748083;-0.0003 -1.22840202974745e-09 490233.705051338 -602180.464147169;-0.000225 -1.25752571484909e-09 507061.746890683 -588080.560696886;-0.00015 -1.28564415313507e-09 523484.451327869 -573510.554644316;-7.5e-05 -1.31273486715606e-09 539488.690304243 -558482.093029369]  x2=[-0.000675 5.43137097459528e-10 369322.642211844 -697989.57461075;-0.0006 5.23109448259394e-10 388907.582416714 -687269.594638426;-0.000525 5.02663633370164e-10 408181.635850686 -676000.221867726;-0.00045 4.81815996863429e-10 427129.395130347 -664190.464862815;-0.000375 4.60583204020834e-10 445735.71370684 -651849.764162748;-0.0003 4.38982228012103e-10 463985.717973781 -638987.984734845;-0.000225 4.17030336326953e-10 481864.819156992 -625615.408088788;-0.00015 3.94745076971722e-10 499358.724976549 -611742.724057743;-7.5e-05 3.72144264441761e-10 516453.451071804 -597381.022253063]  x3=[-0.000675 -6.52487747818041e-14 1409.06764659103 -5515.47701855171;-0.0006 2.88361999804312e-13 1564.42956176397 -5473.43717855314;-0.000525 6.41742262219871e-13 1718.54089588182 -5427.02195662045;-0.00045 9.94609525689999e-13 1871.27845470206 -5376.26845637184;-0.000375 1.34668171352332e-12 2022.52014215712 -5321.21724937888;-0.0003 1.69767738459978e-12 2172.14505795614 -5261.91234273413;-0.000225 2.04731595835032e-12 2320.03359423077 -5198.40114387254;-0.00015 2.39531793904875e-12 2466.06753114787 -5130.73442267476;-7.5e-05 2.74140513923629e-12 2610.13013141267 -5058.96627088235]  x4=[-0.000675 3.37284070319427e-12 5928.29142347721 -10182.4197288333;-0.0006 2.55941471601515e-12 6213.785109469 -10010.7531725406;-0.000525 1.74394277187241e-12 6494.31159071839 -9831.08417333143;-0.00045 9.27076746561042e-13 6769.64661864845 -9643.55635585473;-0.000375 1.09469630283229e-13 7039.57009465063 -9448.31962697853;-0.0003 -7.08224994342091e-13 7303.86624602819 -9245.53005595665;-0.000225 -1.52535347474314e-12 7562.32379848157 -9035.3497496694;-0.00015 -2.34126261091517e-12 7814.73614499788 -8817.94672303775;-7.5e-05 -3.15530017757855e-12 8060.90151100935 -8593.49476471481]  x5=0.000667339049054976  V1=ones(3,3)  V2=ones(3,3)  I1=ones(3,3)  I2=ones(3,3)  nHarmo=1  Measurements=None  Decoupling=off  VsMag0=[ 1 1 1]  VrMag0=[ 1 1 1]  VsAngle0=[0 -120 120]  VrAngle0=[0 -120 120]  IsMag0=[ 1 1 1]  IrMag0=[ 1 1 1]  IsAngle0=[0 -120 120]  IrAngle0=[0 -120 120]
      settings: AttributesFormatString=\n  LibrarySourceBlock=sps_lib/Power Grid Elements/Distributed Parameters Line
  LMO 330 Mvar : spsThreePhaseSeriesRLCLoadLib/Three-Phase Series RLC Load  LConnTagsString=A|B|C  Configuration=Y (grounded)  NominalVoltage=735e3  Vabc=[1e3 1e3 1e3]  Vabcp=[1e3 1e3 1e3]  NominalFrequency=60  UnbalancedPower=off  ActivePower=1100000  InductivePower=330e6  CapacitivePower=0  Pabc=[10e3 9e3 11e3]  QLabc=[100 90 110]  QCabc=[100 90 110]  Pabcp=[10e3 9e3 11e3]  QLabcp=[100 90 110]  QCabcp=[100 90 110]  Measurements=None  LoadType=constant Z
  LMO-ALB 3*218km : spsDistributedParametersLineLib/Distributed Parameters Line  Phases=3  Length=218  Frequency=60  Resistance="[0.01273  0.3864]/3"  Inductance="[0.9337e-3  4.1264e-3]/3"  Capacitance=[12.74e-9 7.751e-9]*3  x1=[-0.001275 6.86459129721463e-10 0 0;-0.0012 6.70322463993873e-10 0 0;-0.001125 6.53649952744844e-10 0 0;-0.00105 6.3645492372477e-10 0 0;-0.000975 6.18751122376757e-10 0 0;-0.0009 6.00552700848726e-10 0 0;-0.000825 5.81874206680401e-10 329282.96109861 -717747.524634827;-0.00075 5.6273057117423e-10 349442.471137616 -708151.592396728;-0.000675 5.43137097459528e-10 369322.642211844 -697989.57461075;-0.0006 5.23109448259394e-10 388907.582416714 -687269.594638426;-0.000525 5.02663633370164e-10 408181.635850686 -676000.221867726;-0.00045 4.81815996863429e-10 427129.395130347 -664190.464862815;-0.000375 4.60583204020834e-10 445735.71370684 -651849.764162748;-0.0003 4.38982228012103e-10 463985.717973781 -638987.984734845;-0.000225 4.17030336326953e-10 481864.819156992 -625615.408088788;-0.00015 3.94745076971722e-10 499358.724976549 -611742.724057743;-7.5e-05 3.72144264441761e-10 516453.451071804 -597381.022253063]  x2=[-0.001275 2.12307559660001e-09 0 0;-0.0012 2.18507452782085e-09 0 0;-0.001125 2.2453267438969e-09 0 0;-0.00105 2.30378408012854e-09 0 0;-0.000975 2.36039980661559e-09 0 0;-0.0009 2.41512866561257e-09 0 0;-0.000825 2.46792690770697e-09 208359.206060615 -779372.311347969;-0.00075 2.51875232679189e-09 230309.218727236 -773170.335952848;-0.000675 2.56756429380498e-09 252075.125728256 -766350.300021069;-0.0006 2.61432378920665e-09 273639.527730648 -758917.655385007;-0.000525 2.65899343417172e-09 294985.186481397 -750878.343587059;-0.00045 2.70153752046948e-09 316095.038587497 -742238.791130071;-0.000375 2.74192203900829e-09 336952.209156166 -733005.904340088;-0.0003 2.78011470702193e-09 357540.025284378 -723187.063845543;-0.000225 2.81608499387596e-09 377842.029386924 -712790.118677292;-0.00015 2.84980414547342e-09 397841.992352354 -701823.379994225;-7.5e-05 2.88124520724047e-09 417523.926516285 -690295.614439449]  x3=[-0.001275 -1.65176885362165e-11 0 0;-0.0012 -1.61011094199933e-11 0 0;-0.001125 -1.5671659323255e-11 0 0;-0.00105 -1.52296815418382e-11 0 0;-0.000975 -1.47755293860187e-11 0 0;-0.0009 -1.43095658980812e-11 0 0;-0.000825 -1.38321635621085e-11 -103.698287433156 -3735.8630713006;-0.00075 -1.33437040062235e-11 1.95817417263447 -3737.30097845969;-0.000675 -1.28445776975213e-11 107.613070443953 -3735.75134439921;-0.0006 -1.23351836299365e-11 213.181942473293 -3731.21540787294;-0.000525 -1.18159290052925e-11 318.580400119613 -3723.69679483912;-0.00045 -1.12872289077914e-11 423.724189468521 -3713.20151556198;-0.000375 -1.07495059722018e-11 528.529260183565 -3699.73795980719;-0.0003 -1.0203190046011e-11 632.911832694788 -3683.31689013522;-0.000225 -9.64871784581152e-12 736.78846517083 -3663.95143329791;-0.00015 -9.08653260819639e-12 840.076120221056 -3641.65706974516;-7.5e-05 -8.51708373544287e-12 942.692231274374 -3616.45162125008]  x4=[-0.001275 2.43205417999027e-11 0 0;-0.0012 2.40945632557638e-11 0 0;-0.001125 2.38493238864175e-11 0 0;-0.00105 2.35850197324633e-11 0 0;-0.000975 2.33018620745979e-11 0 0;-0.0009 2.30000772647205e-11 0 0;-0.000825 2.26799065449906e-11 3660.66083936966 -13572.4875623729;-0.00075 2.23416058549829e-11 4042.89932356971 -13463.5735253601;-0.000675 2.19854456270928e-11 4421.90597590894 -13343.8969136707;-0.0006 2.16117105703569e-11 4797.37782426846 -13213.553394957;-0.000525 2.12206994428614e-11 5169.0147221976 -13072.6471638335;-0.00045 2.08127248129188e-11 5536.51958884639 -12921.2908585854;-0.000375 2.03881128092061e-11 5899.59864644744 -12759.6054711274;-0.0003 1.99472028600624e-11 6257.96165515742 -12587.7202502842;-0.000225 1.94903474221547e-11 6611.32214507028 -12405.7725984716;-0.00015 1.90179116987301e-11 6959.397645217 -12213.9079618584;-7.5e-05 1.85302733476774e-11 7301.90990936848 -12012.2797140996]  x5=0.00123288061605072  V1=ones(3,3)  V2=ones(3,3)  I1=ones(3,3)  I2=ones(3,3)  nHarmo=1  Measurements=None  Decoupling=off  VsMag0=[ 1 1 1]  VrMag0=[ 1 1 1]  VsAngle0=[0 -120 120]  VrAngle0=[0 -120 120]  IsMag0=[ 1 1 1]  IrMag0=[ 1 1 1]  IsAngle0=[0 -120 120]  IrAngle0=[0 -120 120]
      settings: AttributesFormatString=\n  LibrarySourceBlock=sps_lib/Power Grid Elements/Distributed Parameters Line
  LMO7 : spsThreePhaseVIMeasurementLib/Three-Phase V-I Measurement  VoltageMeasurement=no  SetLabelV=on  LabelV=Vabc_LMO7  Vpu=on  VpuLL=off  CurrentMeasurement=no  SetLabelI=off  LabelI=A1  Ipu=off  Pbase=100e6  Vbase=735e3  OutputType=Magnitude  PhasorSimulation=off  PSBequivalent=0
  LVD 990 Mvar : spsThreePhaseSeriesRLCLoadLib/Three-Phase Series RLC Load  LConnTagsString=A|B|C  Configuration=Y (grounded)  NominalVoltage=735e3  Vabc=[1e3 1e3 1e3]  Vabcp=[1e3 1e3 1e3]  NominalFrequency=60  UnbalancedPower=off  ActivePower=3300000  InductivePower=990e6  CapacitivePower=0  Pabc=[10e3 9e3 11e3]  QLabc=[100 90 110]  QCabc=[100 90 110]  Pabcp=[10e3 9e3 11e3]  QLabcp=[100 90 110]  QCabcp=[100 90 110]  Measurements=None  LoadType=constant Z
  LVD-MTL 3*260km : spsDistributedParametersLineLib/Distributed Parameters Line  Phases=3  Length=260  Frequency=60  Resistance="[0.01273  0.3864]/3"  Inductance="[0.9337e-3  4.1264e-3]/3"  Capacitance=[12.74e-9 7.751e-9]*3  x1=[-0.0015 7.97115934916426e-09 -149994.752694816 -815900.545010743;-0.001425 8.12267805978441e-09 -126868.831368404 -819814.854171661;-0.00135 8.26770362584472e-09 -103641.493039354 -823073.815881742;-0.001275 8.40612011612663e-09 -80331.3052865369 -825674.824976859;-0.0012 8.53781688260566e-09 -56956.9019173837 -827615.802250139;-0.001125 8.66268864890172e-09 -33536.9680723075 -828895.196114045;-0.00105 8.78063559443543e-09 -10090.2252880872 -829511.9838407;-0.000975 8.89156343422317e-09 13364.5834678428 -829465.672379432;-0.0009 8.99538349424708e-09 36808.7087802336 -828756.298750914;-0.000825 9.09201278233966e-09 60223.4097740176 -827384.430017571;-0.00075 9.18137405452651e-09 83589.9690954773 -825351.162830279;-0.000675 9.26339587677391e-09 106889.707874612 -822658.122551716;-0.0006 9.33801268209212e-09 130104.000656738 -819307.461957076;-0.000525 9.40516482294865e-09 153214.290291398 -815301.859513173;-0.00045 9.46479861894956e-09 176202.102766656 -810644.517237312;-0.000375 9.51686639975076e-09 199049.061976944 -805339.158137648;-0.0003 9.56132654316493e-09 221736.904412642 -799390.023237071;-0.000225 9.59814350843371e-09 244247.49375964 -792801.868182996;-0.00015 9.62728786463836e-09 266562.835397238 -785579.959445771;-7.5e-05 9.64873631422646e-09 288665.090782769 -777730.070108741]  x2=[-0.0015 1.27974285721043e-08 -353353.509255366 -707507.476280008;-0.001425 1.30053466259217e-08 -333210.629182265 -717214.190537946;-0.00135 1.32028684046349e-08 -312801.38563049 -726347.574745714;-0.001275 1.33898360123561e-08 -292142.093437063 -734900.32781572;-0.0012 1.35660999900404e-08 -271249.267324067 -742865.612808023;-0.001125 1.37315194349609e-08 -250139.608697025 -750237.062395671;-0.00105 1.38859621133444e-08 -228829.992294054 -757008.783954653;-0.000975 1.40293045660769e-08 -207337.452696461 -763175.364274364;-0.0009 1.41614322073947e-08 -185679.170711551 -768731.873884849;-0.000825 1.42822394164832e-08 -163872.45963856 -773673.870997342;-0.00075 1.43916296219077e-08 -141934.751428668 -777997.405054968;-0.000675 1.44895153788118e-08 -119883.582750158 -781699.019890751;-0.0006 1.45758184388191e-08 -97736.5809698775 -784775.75649043;-0.000525 1.46504698125839e-08 -75511.4500621897 -787225.155357843;-0.00045 1.47134098249402e-08 -53225.9564566862 -789045.258481011;-0.000375 1.47645881626052e-08 -30897.9148359756 -790234.610897347;-0.0003 1.48039639143987e-08 -8545.17389489908 -790792.261856726;-0.000225 1.48315056039474e-08 13814.3979274434 -790717.765581505;-0.00015 1.48471912148459e-08 36162.9267314502 -790011.181622865;-7.5e-05 1.48510082082568e-08 58482.5474451391 -788673.074813212]  x3=[-0.0015 1.61072768498755e-11 176.513539924861 -1804.55713842505;-0.001425 1.77684713881383e-11 227.459268206806 -1798.84517601367;-0.00135 1.94154620822401e-11 278.223169029989 -1791.69524429184;-0.001275 2.10469323530198e-11 328.764662508807 -1783.11305880558;-0.0012 2.26615780281055e-11 379.043346546684 -1773.10548002265;-0.001125 2.42581083844492e-11 429.019029132889 -1761.68050784842;-0.00105 2.5835247180112e-11 478.651760471416 -1748.84727523083;-0.000975 2.73917336744714e-11 527.90186491624 -1734.61604085968;-0.0009 2.89263236360391e-11 576.729972687419 -1718.99818096599;-0.000825 3.04377903370797e-11 625.097051342696 -1702.00618022798;-0.00075 3.19249255342387e-11 672.964436979436 -1683.65362179107;-0.000675 3.33865404343934e-11 720.293865141956 -1663.95517640966;-0.0006 3.4821466644956e-11 767.047501409546 -1642.9265907196;-0.000525 3.62285571078689e-11 813.18797164073 -1620.58467465053;-0.00045 3.76066870165453e-11 858.678391849578 -1596.94728798833;-0.000375 3.89547547150222e-11 903.482397690201 -1572.03332609822;-0.0003 4.02716825786078e-11 947.564173525855 -1545.86270482015;-0.000225 4.15564178753174e-11 990.888481059411 -1518.45634454834;-0.00015 4.28079336074119e-11 1033.42068750231 -1489.83615350785;-7.5e-05 4.40252293323641e-11 1075.12679325949 -1460.02501024151]  x4=[-0.0015 4.67527983295145e-11 -8566.49009752852 -13975.6180438593;-0.001425 4.68014119019859e-11 -8167.96786664886 -14212.2119177598;-0.00135 4.68126131418685e-11 -7762.9162872307 -14437.4447669074;-0.001275 4.67863930950625e-11 -7351.65915130913 -14651.1365436086;-0.0012 4.67227727214722e-11 -6934.52521154617 -14853.1164259268;-0.001125 4.66218028782506e-11 -6511.84791843088 -15043.2229542344;-0.00105 4.64835642791457e-11 -6083.96515372422 -15221.3041602814;-0.000975 4.63081674299784e-11 -5651.21896036146 -15387.2176886764;-0.0009 4.60957525403064e-11 -5213.95526902833 -15540.8309106834;-0.000825 4.58464894113423e-11 -4772.52362162934 -15682.0210302432;-0.00075 4.55605773002175e-11 -4327.27689186927 -15810.6751821343;-0.000675 4.52382447606992e-11 -3878.57100317141 -15926.6905221962;-0.0006 4.48797494604875e-11 -3426.76464415773 -16029.9743095413;-0.000525 4.44853779752403e-11 -2972.21898191877 -16120.4439806901;-0.00045 4.40554455594888e-11 -2515.29737330214 -16198.0272155718;-0.000375 4.3590295894628e-11 -2056.36507445063 -16262.6619953356;-0.0003 4.30903008141829e-11 -1595.78894882205 -16314.2966519273;-0.000225 4.25558600065706e-11 -1133.93717392416 -16352.8899093926;-0.00015 4.19874006955956e-11 -671.178946999267 -16378.4109168719;-7.5e-05 4.13853772989333e-11 -207.884189893521 -16390.8392732624]  x5=0.00147040807418893  V1=ones(3,3)  V2=ones(3,3)  I1=ones(3,3)  I2=ones(3,3)  nHarmo=1  Measurements=None  Decoupling=off  VsMag0=[ 1 1 1]  VrMag0=[ 1 1 1]  VsAngle0=[0 -120 120]  VrAngle0=[0 -120 120]  IsMag0=[ 1 1 1]  IrMag0=[ 1 1 1]  IsAngle0=[0 -120 120]  IrAngle0=[0 -120 120]
      settings: AttributesFormatString=\n  LibrarySourceBlock=sps_lib/Power Grid Elements/Distributed Parameters Line
  LVD7 : spsThreePhaseVIMeasurementLib/Three-Phase V-I Measurement  VoltageMeasurement=no  SetLabelV=on  LabelV=Vabc_LVD7  Vpu=on  VpuLL=off  CurrentMeasurement=no  SetLabelI=off  LabelI=A1  Ipu=off  Pbase=100e6  Vbase=735e3  OutputType=Magnitude  PhasorSimulation=off  PSBequivalent=0
  Load Flow Bus1 : spsLoadFlowBusLib/Load Flow Bus  LConnTagsString=a  Phases=single  Connectors=on one side  ID=LG31_13.8  Vbase=13.8e3  Vref=1  Vangle=0  VLF=1  VLFb=1  VLFc=1  angleLF=-0.0351  angleLFb=0  angleLFc=0
      settings: AttributesFormatString=%<ID>\n%<Vbase>V\n%<VLF>pu\n%<angleLF>deg.
  Load Flow Bus10 : spsLoadFlowBusLib/Load Flow Bus  LConnTagsString=a  Phases=single  Connectors=on one side  ID=LVD7  Vbase=735e3  Vref=1  Vangle=0  VLF=1.05  VLFb=1  VLFc=1  angleLF=-12.02  angleLFb=0  angleLFc=0
      settings: AttributesFormatString=%<ID>\n%<Vbase>V\n%<VLF>pu\n%<angleLF>deg.
  Load Flow Bus11 : spsLoadFlowBusLib/Load Flow Bus  LConnTagsString=a  Phases=single  Connectors=on one side  ID=CHM7  Vbase=735e3  Vref=1  Vangle=0  VLF=1.047  VLFb=1  VLFc=1  angleLF=-4.064  angleLFb=0  angleLFc=0
      settings: AttributesFormatString=%<ID>\n%<Vbase>V\n%<VLF>pu\n%<angleLF>deg.
  Load Flow Bus12 : spsLoadFlowBusLib/Load Flow Bus  LConnTagsString=a  Phases=single  Connectors=on one side  ID=LG47  Vbase=735e3  Vref=1  Vangle=0  VLF=1.004  VLFb=1  VLFc=1  angleLF=20.71  angleLFb=0  angleLFc=0
      settings: AttributesFormatString=%<ID>\n%<Vbase>V\n%<VLF>pu\n%<angleLF>deg.
  Load Flow Bus2 : spsLoadFlowBusLib/Load Flow Bus  LConnTagsString=a  Phases=single  Connectors=on one side  ID=LG3_13.8  Vbase=13.8e3  Vref=1  Vangle=0  VLF=1  VLFb=1  VLFc=1  angleLF=-0.6025  angleLFb=0  angleLFc=0
      settings: AttributesFormatString=%<ID>\n%<Vbase>V\n%<VLF>pu\n%<angleLF>deg.
  Load Flow Bus3 : spsLoadFlowBusLib/Load Flow Bus  LConnTagsString=a  Phases=single  Connectors=on one side  ID=LG4_13.8  Vbase=13.8e3  Vref=1  Vangle=0  VLF=1  VLFb=1  VLFc=1  angleLF=-3.293  angleLFb=0  angleLFc=0
      settings: AttributesFormatString=%<ID>\n%<Vbase>V\n%<VLF>pu\n%<angleLF>deg.
  Load Flow Bus4 : spsLoadFlowBusLib/Load Flow Bus  LConnTagsString=a  Phases=single  Connectors=on one side  ID=LG2_13.8  Vbase=13.8e3  Vref=1  Vangle=0  VLF=1  VLFb=1  VLFc=1  angleLF=0  angleLFb=0  angleLFc=0
      settings: AttributesFormatString=%<ID>\n%<Vbase>V\n%<VLF>pu\n%<angleLF>deg.
  Load Flow Bus5 : spsLoadFlowBusLib/Load Flow Bus  LConnTagsString=a  Phases=single  Connectors=on one side  ID=LG27  Vbase=735e3  Vref=1  Vangle=0  VLF=1  VLFb=1  VLFc=1  angleLF=23.57  angleLFb=0  angleLFc=0
      settings: AttributesFormatString=%<ID>\n%<Vbase>V\n%<VLF>pu\n%<angleLF>deg.
  Load Flow Bus6 : spsLoadFlowBusLib/Load Flow Bus  LConnTagsString=a  Phases=single  Connectors=on one side  ID=LG37  Vbase=735e3  Vref=1  Vangle=0  VLF=0.994  VLFb=1  VLFc=1  angleLF=24.1  angleLFb=0  angleLFc=0
      settings: AttributesFormatString=%<ID>\n%<Vbase>V\n%<VLF>pu\n%<angleLF>deg.
  Load Flow Bus7 : spsLoadFlowBusLib/Load Flow Bus  LConnTagsString=a  Phases=single  Connectors=on one side  ID=LMO7  Vbase=735e3  Vref=1  Vangle=0  VLF=1.016  VLFb=1  VLFc=1  angleLF=17.31  angleLFb=0  angleLFc=0
      settings: AttributesFormatString=%<ID>\n%<Vbase>V\n%<VLF>pu\n%<angleLF>deg.
  Load Flow Bus8 : spsLoadFlowBusLib/Load Flow Bus  LConnTagsString=a  Phases=single  Connectors=on one side  ID=NEM_ALB7  Vbase=735e3  Vref=1  Vangle=0  VLF=1.028  VLFb=1  VLFc=1  angleLF=8.928  angleLFb=0  angleLFc=0
      settings: AttributesFormatString=%<ID>\n%<Vbase>V\n%<VLF>pu\n%<angleLF>deg.
  Load Flow Bus9 : spsLoadFlowBusLib/Load Flow Bus  LConnTagsString=a  Phases=single  Connectors=on one side  ID=ABI_CHB7  Vbase=735e3  Vref=1  Vangle=0  VLF=1.046  VLFb=1  VLFc=1  angleLF=0.1334  angleLFb=0  angleLFc=0
      settings: AttributesFormatString=%<ID>\n%<Vbase>V\n%<VLF>pu\n%<angleLF>deg.
  NEM-ABI 6*236 : spsDistributedParametersLineLib/Distributed Parameters Line  Phases=3  Length=236  Frequency=60  Resistance="[0.01273  0.3864]/6"  Inductance="[0.9337e-3  4.1264e-3]/6"  Capacitance=[12.74e-9 7.751e-9]*6  x1=[-0.00135 1.98718245820778e-09 0 0;-0.001275 2.03092470403277e-09 0 0;-0.0012 2.07304345972355e-09 0 0;-0.001125 2.11350505619126e-09 0 0;-0.00105 2.15227714905476e-09 0 0;-0.000975 2.18932874449624e-09 0 0;-0.0009 2.22463022403723e-09 0 0;-0.000825 2.25815336821511e-09 235173.136251957 -772031.417007292;-0.00075 2.28987137914134e-09 256904.899781926 -765074.329412273;-0.000675 2.3197589019233e-09 278431.297465786 -757505.653104351;-0.0006 2.34779204493256e-09 299735.121430593 -749331.438367563;-0.000525 2.37394839890352e-09 320799.34172543 -740558.219544099;-0.00045 2.39820705484702e-09 341607.119934886 -731193.009810853;-0.000375 2.42054862076468e-09 362141.82263943 -721243.295573192;-0.0003 2.44095523715054e-09 382387.034711912 -710717.030480442;-0.000225 2.45941059126769e-09 402326.572439563 -699622.629067861;-0.00015 2.47589993018842e-09 421944.496461009 -687968.960030189;-7.5e-05 2.4904100725875e-09 441225.124507952 -675765.339132147]  x2=[-0.00135 4.03348351098424e-09 0 0;-0.001275 4.12470348880822e-09 0 0;-0.0012 4.21262624177332e-09 0 0;-0.001125 4.29718148577609e-09 0 0;-0.00105 4.37830162864821e-09 0 0;-0.000975 4.45592182418866e-09 0 0;-0.0009 4.52998002400073e-09 0 0;-0.000825 4.60041702709264e-09 81706.5138319585 -820341.457427458;-0.00075 4.66717652720183e-09 104865.377019367 -817703.66746532;-0.000675 4.73020515780538e-09 127940.412428881 -814412.217702696;-0.0006 4.78945253478034e-09 150913.174230253 -810469.739274165;-0.000525 4.84487129668007e-09 173765.298349194 -805879.383736661;-0.00045 4.89641714259426e-09 196478.517147333 -800644.820550167;-0.000375 4.94404886756235e-09 219034.674025087 -794770.234144401;-0.0003 4.9877283955122e-09 241415.737935768 -788260.320573852;-0.000225 5.02742080969748e-09 263603.817799327 -781120.283763824;-0.00015 5.0630943806096e-09 285581.176804212 -773355.831350496;-7.5e-05 5.09472059134181e-09 307330.246585898 -764973.170118328]  x3=[-0.00135 4.15195616424837e-13 0 0;-0.001275 2.00507645006235e-12 0 0;-0.0012 3.59335445626438e-12 0 0;-0.001125 5.17875998989424e-12 0 0;-0.00105 6.76002570202586e-12 0 0;-0.000975 8.33588755304315e-12 0 0;-0.0009 9.90508582309389e-12 0 0;-0.000825 1.14663661190905e-11 -1379.76964293767 -6710.39772290078;-0.00075 1.30184803774529e-11 -1189.51028635371 -6746.72121821219;-0.000675 1.45601878617909e-11 -998.300053446964 -6777.65148781004;-0.0006 1.60902561547306e-11 -806.291794751993 -6803.16380651009;-0.000525 1.76074621430893e-11 -613.638998732974 -6823.23778015512;-0.00045 1.91105929956141e-11 -420.49566908736 -6837.85736191772;-0.000375 2.05984471325e-11 -227.016201637677 -6847.01086512793;-0.0003 2.2069835185915e-11 -33.3552609098692 -6850.69097261534;-0.000225 2.35235809507623e-11 160.332343503157 -6848.89474255833;-0.00015 2.49585223249203e-11 353.891780693955 -6841.62361083572;-7.5e-05 2.637351223821e-11 547.168322209991 -6828.88338987896]  x4=[-0.00135 3.52882273313557e-11 0 0;-0.001275 3.49733195135572e-11 0 0;-0.0012 3.46304545592493e-11 0 0;-0.001125 3.42599065494305e-11 0 0;-0.00105 3.38619716945102e-11 0 0;-0.000975 3.34369680975229e-11 0 0;-0.0009 3.29852354998412e-11 0 0;-0.000825 3.25071350095919e-11 2916.74328192661 -29367.0114378;-0.00075 3.20030488129918e-11 3745.79818278436 -29272.8158501747;-0.000675 3.14733798688337e-11 4571.85874988742 -29155.220021448;-0.0006 3.09185515863673e-11 5394.26464305761 -29014.317955926;-0.000525 3.03390074868325e-11 6212.35844360716 -28850.2222885639;-0.00045 2.9735210848915e-11 7025.48617986915 -28663.0641949275;-0.000375 2.91076443384089e-11 7832.99784997251 -28452.9932863333;-0.0003 2.84568096223806e-11 8634.24794144348 -28220.1774902515;-0.000225 2.7783226968144e-11 9428.59594721848 -27964.8029160671;-0.00015 2.70874348273666e-11 10215.4068776556 -27687.0737063074;-7.5e-05 2.63699894056399e-11 10994.0517681358 -27387.2118734533]  x5=0.00133467809810995  V1=ones(3,3)  V2=ones(3,3)  I1=ones(3,3)  I2=ones(3,3)  nHarmo=1  Measurements=None  Decoupling=off  VsMag0=[ 1 1 1]  VrMag0=[ 1 1 1]  VsAngle0=[0 -120 120]  VrAngle0=[0 -120 120]  IsMag0=[ 1 1 1]  IrMag0=[ 1 1 1]  IsAngle0=[0 -120 120]  IrAngle0=[0 -120 120]
      settings: AttributesFormatString=\n  LibrarySourceBlock=sps_lib/Power Grid Elements/Distributed Parameters Line
  NEM-ALB 1980 Mvar : spsThreePhaseSeriesRLCLoadLib/Three-Phase Series RLC Load  LConnTagsString=A|B|C  Configuration=Y (grounded)  NominalVoltage=735e3  Vabc=[1e3 1e3 1e3]  Vabcp=[1e3 1e3 1e3]  NominalFrequency=60  UnbalancedPower=off  ActivePower=6600000  InductivePower=1980e6  CapacitivePower=0  Pabc=[10e3 9e3 11e3]  QLabc=[100 90 110]  QCabc=[100 90 110]  Pabcp=[10e3 9e3 11e3]  QLabcp=[100 90 110]  QCabcp=[100 90 110]  Measurements=None  LoadType=constant Z
  NEM-ALB7 : spsThreePhaseVIMeasurementLib/Three-Phase V-I Measurement  VoltageMeasurement=no  SetLabelV=on  LabelV=Vabc_NEM7  Vpu=on  VpuLL=off  CurrentMeasurement=no  SetLabelI=off  LabelI=A1  Ipu=off  Pbase=100e6  Vbase=735e3  OutputType=Magnitude  PhasorSimulation=off  PSBequivalent=0
  Regulators1 : Subsystem
  Regulators2 : Subsystem
  Regulators3 : Subsystem
  Regulators4 : Subsystem
  MTLa : PMIOPort  Side=Right
  MTLb : PMIOPort  Port=2  Side=Right
  MTLc : PMIOPort  Port=3  Side=Right
  CHM7a : PMIOPort  Port=4  Side=Right
  CHM7b : PMIOPort  Port=5  Side=Right
  CHM7c : PMIOPort  Port=6  Side=Right
  wires:
  Regulators2/1(Pm) -> LG3_2200 MVA/1
  Regulators4/2(Vf) -> LG4-2700 MVA/2
  Regulators4/1(Pm) -> LG4-2700 MVA/1
  Regulators3/2(Vf) -> LG31-200 MVA/2
  Regulators3/1(Pm) -> LG31-200 MVA/1
  Regulators2/2(Vf) -> LG3_2200 MVA/2
  LG3_2200 MVA/1 -> Regulators2/1(m)
  Regulators1/1(Pm) -> LG2_5500 MVA/1
  Regulators1/2(Vf) -> LG2_5500 MVA/2
  LG2_5500 MVA/1 -> Regulators1/1(m)
  LG31-200 MVA/1 -> Regulators3/1(m)
  LG4-2700 MVA/1 -> Regulators4/1(m)
  connections:
  LG2-NENI 3*279km/RConn1 -- "Cs NEM "/LConn1
  LG2-NENI 3*279km/RConn2 -- "Cs NEM "/LConn2
  LG2-NENI 3*279km/RConn3 -- "Cs NEM "/LConn3
  CHB-CHM 3*195km/RConn1 -- "Cs  CHMN "/LConn1
  CHB-CHM 3*195km/RConn2 -- "Cs  CHMN "/LConn2
  CHB-CHM 3*195km/RConn3 -- "Cs  CHMN "/LConn3
  Load Flow Bus2/LConn1 -- 2200 MVA 13.8 kV/735 kV/LConn1 -- LG3_2200 MVA/RConn1 -- 110 MW/LConn1
  2200 MVA 13.8 kV/735 kV/LConn2 -- LG3_2200 MVA/RConn2 -- 110 MW/LConn2
  2200 MVA 13.8 kV/735 kV/LConn3 -- LG3_2200 MVA/RConn3 -- 110 MW/LConn3
  Load Flow Bus1/LConn1 -- 200 MVA 13.8 kV/735 kV/LConn1 -- LG31-200 MVA/RConn1 -- 10 MW/LConn1
  200 MVA 13.8 kV/735 kV/LConn2 -- LG31-200 MVA/RConn2 -- 10 MW/LConn2
  200 MVA 13.8 kV/735 kV/LConn3 -- LG31-200 MVA/RConn3 -- 10 MW/LConn3
  Load Flow Bus6/LConn1 -- 2200 MVA 13.8 kV/735 kV/RConn1 -- 200 MVA 13.8 kV/735 kV/RConn1 -- LG3-LMO 104km/LConn1 -- LG3 660 Mvar/LConn1 -- LG2-LG3 155km/RConn1
  2200 MVA 13.8 kV/735 kV/RConn2 -- LG3 660 Mvar/LConn2 -- LG2-LG3 155km/RConn2 -- 200 MVA 13.8 kV/735 kV/RConn2 -- LG3-LMO 104km/LConn2
  LG3-LMO 104km/RConn1 -- LMO7/RConn1 -- LG4-LMO 3*118km/RConn1 -- LMO 330 Mvar/LConn1
  LG3-LMO 104km/RConn2 -- LMO7/RConn2 -- LG4-LMO 3*118km/RConn2 -- LMO 330 Mvar/LConn2
  LG3-LMO 104km/RConn3 -- LMO7/RConn3 -- LG4-LMO 3*118km/RConn3 -- LMO 330 Mvar/LConn3
  LG4-LMO 3*118km/LConn1 -- LG4 660 Mvar/LConn1 -- 2700 MVA 13.8 kV/735 kV/RConn1 -- Load Flow Bus12/LConn1
  LG4-LMO 3*118km/LConn2 -- 2700 MVA 13.8 kV/735 kV/RConn2 -- LG4 660 Mvar/LConn2
  LG4 660 Mvar/LConn3 -- 2700 MVA 13.8 kV/735 kV/RConn3 -- LG4-LMO 3*118km/LConn3
  Load Flow Bus3/LConn1 -- LG4-2700 MVA/RConn1 -- 2700 MVA 13.8 kV/735 kV/LConn1 -- 135 MW/LConn1
  LG4-2700 MVA/RConn2 -- 2700 MVA 13.8 kV/735 kV/LConn2 -- 135 MW/LConn2
  LG4-2700 MVA/RConn3 -- 2700 MVA 13.8 kV/735 kV/LConn3 -- 135 MW/LConn3
  Load Flow Bus4/LConn1 -- 5500 MVA 13.8 kV/735 kV/LConn1 -- LG2_5500 MVA/RConn1 -- 275 MW/LConn1
  5500 MVA 13.8 kV/735 kV/LConn2 -- LG2_5500 MVA/RConn2 -- 275 MW/LConn2
  LG2_5500 MVA/RConn3 -- 5500 MVA 13.8 kV/735 kV/LConn3 -- 275 MW/LConn3
  5500 MVA 13.8 kV/735 kV/RConn1 -- LG2-NENI 3*279km/LConn1 -- LG2-LG3 155km/LConn1 -- LG2 660 Mvar/LConn1 -- Load Flow Bus5/LConn1
  LG2-LG3 155km/LConn2 -- 5500 MVA 13.8 kV/735 kV/RConn2 -- LG2-NENI 3*279km/LConn2 -- LG2 660 Mvar/LConn2
  LG2-LG3 155km/LConn3 -- 5500 MVA 13.8 kV/735 kV/RConn3 -- LG2-NENI 3*279km/LConn3 -- LG2 660 Mvar/LConn3
  "Cs NEM "/RConn1 -- NEM-ALB7/LConn1 -- Cs ALB/RConn1
  "Cs NEM "/RConn2 -- NEM-ALB7/LConn2 -- Cs ALB/RConn2
  "Cs NEM "/RConn3 -- NEM-ALB7/LConn3 -- Cs ALB/RConn3
  LMO7/LConn1 -- LMO-ALB 3*218km/LConn1
  LMO7/LConn2 -- LMO-ALB 3*218km/LConn2
  Load Flow Bus7/LConn1 -- LMO7/LConn3 -- LMO-ALB 3*218km/LConn3
  Cs ALB/LConn1 -- LMO-ALB 3*218km/RConn1
  Cs ALB/LConn2 -- LMO-ALB 3*218km/RConn2
  Cs ALB/LConn3 -- LMO-ALB 3*218km/RConn3
  200 MVA 13.8 kV/735 kV/RConn3 -- LG3-LMO 104km/LConn3 -- LG3 660 Mvar/LConn3 -- LG2-LG3 155km/RConn3 -- 2200 MVA 13.8 kV/735 kV/RConn3
  Load Flow Bus8/LConn1 -- NEM-ABI 6*236/LConn1 -- NEM-ALB7/RConn1 -- NEM-ALB 1980 Mvar/LConn1
  NEM-ALB 1980 Mvar/LConn2 -- NEM-ALB7/RConn2 -- NEM-ABI 6*236/LConn2
  NEM-ALB 1980 Mvar/LConn3 -- NEM-ALB7/RConn3 -- NEM-ABI 6*236/LConn3
  NEM-ABI 6*236/RConn1 -- "Cs ABI+CHB "/LConn1
  NEM-ABI 6*236/RConn2 -- "Cs ABI+CHB "/LConn2
  NEM-ABI 6*236/RConn3 -- "Cs ABI+CHB "/LConn3
  "Cs ABI+CHB "/RConn1 -- ABI-CHB7/LConn1
  "Cs ABI+CHB "/RConn2 -- ABI-CHB7/LConn2
  "Cs ABI+CHB "/RConn3 -- ABI-CHB7/LConn3
  Load Flow Bus9/LConn1 -- ABI+CHB 1320 Mvar/LConn1 -- CHB-CHM 3*195km/LConn1 -- ABI-CHB 3*271km/LConn1 -- ABI-CHB7/RConn1
  ABI-CHB 3*271km/LConn2 -- ABI-CHB7/RConn2 -- ABI+CHB 1320 Mvar/LConn2 -- CHB-CHM 3*195km/LConn2
  ABI-CHB 3*271km/LConn3 -- ABI-CHB7/RConn3 -- ABI+CHB 1320 Mvar/LConn3 -- CHB-CHM 3*195km/LConn3
  ABI-CHB 3*271km/RConn1 -- "Cs LVDN "/LConn1
  ABI-CHB 3*271km/RConn2 -- "Cs LVDN "/LConn2
  ABI-CHB 3*271km/RConn3 -- "Cs LVDN "/LConn3
  "Cs LVDN "/RConn1 -- LVD7/LConn1
  "Cs LVDN "/RConn2 -- LVD7/LConn2
  "Cs LVDN "/RConn3 -- LVD7/LConn3
  "Cs LVDS "/LConn1 -- LVD 990 Mvar/LConn1 -- Load Flow Bus10/LConn1 -- LVD7/RConn1
  "Cs LVDS "/LConn2 -- LVD7/RConn2 -- LVD 990 Mvar/LConn2
  "Cs LVDS "/LConn3 -- LVD7/RConn3 -- LVD 990 Mvar/LConn3
  "Cs LVDS "/RConn1 -- LVD-MTL 3*260km/LConn1
  "Cs LVDS "/RConn2 -- LVD-MTL 3*260km/LConn2
  "Cs LVDS "/RConn3 -- LVD-MTL 3*260km/LConn3
  MTLa/RConn1 -- LVD-MTL 3*260km/RConn1
  MTLb/RConn1 -- LVD-MTL 3*260km/RConn2
  MTLc/RConn1 -- LVD-MTL 3*260km/RConn3
  "Cs  CHMN "/RConn1 -- CHM7/LConn1
  "Cs  CHMN "/RConn2 -- CHM7/LConn2
  "Cs  CHMN "/RConn3 -- CHM7/LConn3
  CHM 1320Mvar/LConn2 -- CHM7/RConn2 -- CHM7b/RConn1
  Load Flow Bus11/LConn1 -- CHM 1320Mvar/LConn3 -- CHM7c/RConn1 -- CHM7/RConn3
  CHM7a/RConn1 -- CHM 1320Mvar/LConn1 -- CHM7/RConn1
